simulink subsystem "Subsistema_Mecanico"  (R2023b)
settings: Solver=VariableStepAuto  StartTime=0.0  StopTime=10.0  RelTol=1e-3
values from neighbouring files (symbols this model uses):
  b_eq = b_m + b_l/(r^2)    (= 2.19444444444e-05)    [constantes.m]    (also in test_polos_PID.m = b_m + b_l_nominal/(r^2))
  J_eq = J_m + J_l/(r^2)    (= 1.97847222222e-05)    [constantes.m]    (also in test_polos_PID.m = J_m + J_l/(r^2))
  k_l = g*(m*l_cm + m_l*l_l)    (= 2.4516625)    [constantes.m]
  r = 120    [constantes.m]
settings Model: Creator=rodri  LastModifiedBy=Nahuel

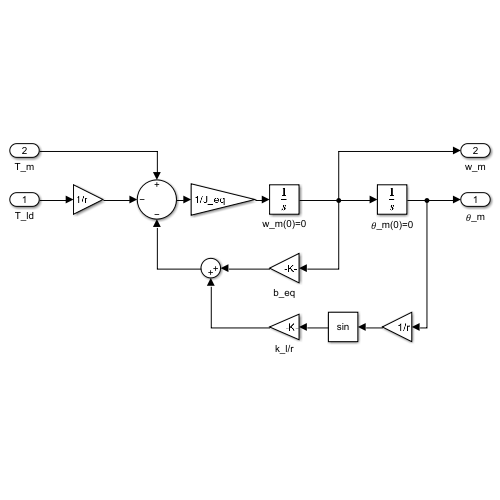
[thumbnail: Simulink's stored preview of the top-level diagram]
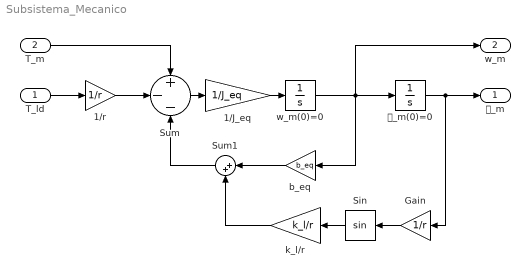
== system Subsistema_Mecanico ==
  T_ld : Inport
  T_m : Inport  Port=2
  1/J_eq : Gain  Gain=1/J_eq
  1/r : Gain  Gain=1/r
  Gain : Gain  Gain=1/r
  Sin : Trigonometry
  Sum : Sum  Inputs=+--
  Sum1 : Sum  Inputs=|++
  b_eq : Gain  Gain=b_eq
  k_l/r : Gain  Gain=k_l/r
  w_m(0)=0 : Integrator
  𝜃_m(0)=0 : Integrator
  "𝜃_m " : Outport
  w_m : Outport  Port=2
  wires:
  T_ld/1 -> 1/r/1
  T_m/1 -> Sum/1
  1/r/1 -> Sum/2
  𝜃_m(0)=0/1 -> "𝜃_m "/1, Gain/1
  w_m(0)=0/1 -> w_m/1, 𝜃_m(0)=0/1, b_eq/1
  Gain/1 -> Sin/1
  Sin/1 -> k_l/r/1
  b_eq/1 -> Sum1/1
  k_l/r/1 -> Sum1/2
  Sum/1 -> 1/J_eq/1
  Sum1/1 -> Sum/3
  1/J_eq/1 -> w_m(0)=0/1
